simulink model "buoyancy_simulation"  (R2025a)
settings: Solver=VariableStepAuto  StartTime=0.0  StopTime=100  RelTol=1e-3
InitFcn:
  | parameters
values from neighbouring files (symbols this model uses):
  area = pi*(d/2)^2    (= 0.00785398163397)    [parameters.m]    (also in simulation_matlab.m)
  density = 1000    [parameters.m]
  gravity = 9.81    [parameters.m]
  km = 50    [parameters.m]
  mass = 3    [parameters.m]
  p = 0.002    [parameters.m]    (also in simulation_matlab.m)
  surface_buoyancy = 2.94    [parameters.m]
libraries: slpidlib x1
settings Model: Creator=hannasennero  LastModifiedBy=hannasennero

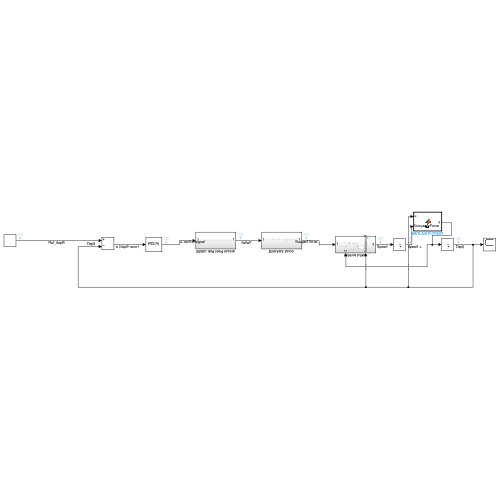
[thumbnail: Simulink's stored preview of the top-level diagram]
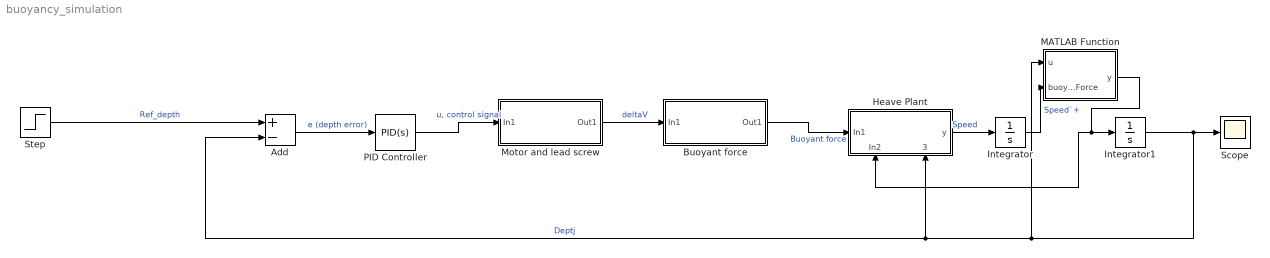
== system buoyancy_simulation ==
  Add : Sum  Inputs=+-
  Buoyant force : Subsystem
  Heave Plant : Subsystem
      settings: PortSchema="{\"entries\":[{\"content\":{\"sides\":[{\"content\":{\"connectorIds\":[\"In1\"]},\"type\":\"ConnectorPlacement.EquallySpacedRectSide\",\"uuid\":\"64163796-67b4-4874-a81c-abb8813ac274\"},{\"content\":{\"connectorIds\":[\"Out1\"],\"side\":\"RIGHT\"},\"type\":\"ConnectorPlacement.EquallySpacedRectSide\",\"uuid\":\"c10edb53-fdb3-4b5f-a96a-74da846fe7c3\"},{\"content\":{\"side\":\"TOP\"},\"type\":\"ConnectorPlacement.EquallySpacedRectSide\",\"uuid\":\"03a8d6bf-bc70-4644-992b-47d9b15e439c\"},{\"content\":{\"connectorIds\":[\"In2\",\"In3\"],\"side\":\"BOTTOM\"},\"type\":\"ConnectorPlacement.EquallySpacedRectSide\",\"uuid\":\"3bbf4b5d-45ae-4ac2-bdf5-5e5dee5a19eb\"}]},\"type\":\"ConnectorPlacement.EquallySpacedConnector\",\"uuid\":\"f3efd6ea-c772-4fc4-945d-e21c2b4b2ad1\"}],\"packageUris\":[\"http://schema.mathworks.com/mf0/Connector/R2020b\"],\"version\":\"1.0\"}"
  Integrator : Integrator
  Integrator1 : Integrator
  MATLAB Function : MATLAB Function  TreatAsAtomicUnit=on
  Motor and lead screw : Subsystem
  PID Controller : slpidlib/PID Controller  Controller=PID  Form=Parallel  TimeDomain=Continuous-time  UseExternalTs=off  SampleTime=-1  IntegratorMethod=Forward Euler  FilterMethod=Forward Euler  ControllerParametersSource=internal  P=5  I=0  UseKiTs=off  D=1  UseExternalDerivativeSource=off  N=100  UseFilter=on  TunerSelectOption=Transfer Function Based (PID Tuner App)  InitialConditionSource=internal  InitialConditionForIntegrator=0  InitialConditionForFilter=0  DifferentiatorICPrevScaledInput=0  ExternalReset=none  TrackingMode=off  Kt=1  LimitOutput=off  SatLimitsSource=internal  UpperSaturationLimit=inf  LowerSaturationLimit=-inf  LinearizeAsGain=on  AntiWindupMode=none  Kb=1  LimitIntegrator=off  UpperIntegratorSaturationLimit=inf  LowerIntegratorSaturationLimit=-inf  POutMin=[]  POutMax=[]  IOutMin=[]  IOutMax=[]  DOutMin=[]  DOutMax=[]  NOutMin=[]  NOutMax=[]  SumOutMin=[]  SumOutMax=[]  SaturationOutMin=[]  SaturationOutMax=[]  PParamMin=[]  PParamMax=[]  IParamMin=[]  IParamMax=[]  DParamMin=[]  DParamMax=[]  NParamMin=[]  NParamMax=[]  KbParamMin=[]  KbParamMax=[]  KtParamMin=[]  KtParamMax=[]  KbOutMin=[]  KbOutMax=[]  KtOutMin=[]  KtOutMax=[]  IntegratorOutMin=[]  IntegratorOutMax=[]  FilterOutMin=[]  FilterOutMax=[]  SumI1OutMin=[]  SumI1OutMax=[]  SumI2OutMin=[]  SumI2OutMax=[]  SumI3OutMin=[]  SumI3OutMax=[]  SumI4OutMin=[]  SumI4OutMax=[]  SumDOutMin=[]  SumDOutMax=[]  DifferentiatorOutMin=[]  DifferentiatorOutMax=[]  FilterDiffOutCoefMin=[]  FilterDiffOutCoefMax=[]  ReciprocalOutMin=[]  ReciprocalOutMax=[]  SumDenOutMin=[]  SumDenOutMax=[]  SumNumOutMin=[]  SumNumOutMax=[]  DivideOutMin=[]  DivideOutMax=[]  UdiffTsProdOutMin=[]  UdiffTsProdOutMax=[]  NTsProdOutMin=[]  NTsProdOutMax=[]  UintegralTsProdOutMin=[]  UintegralTsProdOutMax=[]  UngainTsProdOutMin=[]  UngainTsProdOutMax=[]  ClampingZeroOutDataTypeStr=Inherit: Inherit via back propagation  ClampingZeroOutMin=[]  ClampingZeroOutMax=[]  FilterDenConstantOutDataTypeStr=Inherit: Inherit via back propagation  FilterDenConstantOutMin=[]  FilterDenConstantOutMax=[]  PCopyOutDataTypeStr=Inherit: Inherit via back propagation  PCopyOutMin=[]  PCopyOutMax=[]  NCopyOutDataTypeStr=Inherit: Inherit via back propagation  NCopyOutMin=[]  NCopyOutMax=[]  IntegratorContinuousStateAttributes=''  IntegratorStateMustResolveToSignalObject=off  IntegratorRTWStateStorageClass=Auto  FilterContinuousStateAttributes=''  FilterStateMustResolveToSignalObject=off  FilterRTWStateStorageClass=Auto  ParallelPVariant=InternalParameters  IdealPVariant=Disabled  IVariant=InternalParameters  DVariant=InternalParameters  IntegratorVariant=Continuous  SatVariant=Disabled  AWVariant=Passthrough  PCopyVariant=Disabled  TRVariant=Disabled  FdbkBlocksVariant=Forward  IdealPFdbkVariant=Disabled  SatFdbkVariant=Disabled  DerivativeFilterVariant=ContFilter  NVariant=InternalParameters  NCopyVariant=Disabled  FilterICVariant=InternalICsFilter  IntegratorICVariant=InternalICs  ExternalResetVariant=Disabled  TRSumVariant=Passthrough  SumFdbkVariant=Disabled  SumVariant=Sum_PID  TsampFilterVariant=InternalTs  TsampNgainVariant=Passthrough  TsampIntegralVariant=Disabled_SignalSpec  ExternalSaturationOutDataTypeStr=Inherit: Same as second input  DerivativeSourceVariant=ErrorSignal  PreIntVariant=InternalPreInt
  Scope : Scope
      settings: ActiveDisplayYMinimum=-21.142736439512891  ActiveDisplayYMaximum=-18.092954060228088
  Step : Step  After=-3  SampleTime=0
  wires:
  Step/1 -> Add/1  "Ref_depth"
  Heave Plant/1(y) -> Integrator/1  "Speed"
  Add/1 -> PID Controller/1  "e (depth error)"
  PID Controller/1 -> Motor and lead screw/1(In1)  "u, control signal"
  Motor and lead screw/1(Out1) -> Buoyant force/1(In1)  "deltaV"
  Buoyant force/1(Out1) -> Heave Plant/1(In1)  "Buoyant force"
  Integrator/1 -> MATLAB Function/2(buoyancyForce)  "Speed`+"
  Integrator1/1 -> Scope/1, MATLAB Function/1(u), Heave Plant/3(buoyancyForce), Add/2  "Deptj"
  MATLAB Function/1(y) -> Integrator1/1, Heave Plant/2(In2)

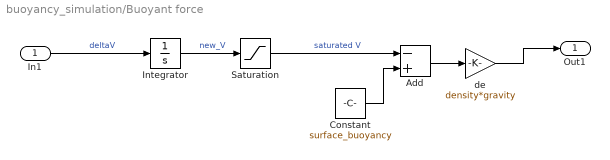
== system buoyancy_simulation/Buoyant force ==
  In1 : Inport
  Add : Sum  Inputs=-+
  Constant : Constant  Value=surface_buoyancy
  Integrator : Integrator
  Saturation : Saturate  UpperLimit=500  LowerLimit=-500
  de : Gain  Gain=density*gravity
  Out1 : Outport
  wires:
  In1/1 -> Integrator/1  "deltaV"
  Integrator/1 -> Saturation/1  "new_V"
  Add/1 -> de/1
  Constant/1 -> Add/2
  Saturation/1 -> Add/1  "saturated V"
  de/1 -> Out1/1

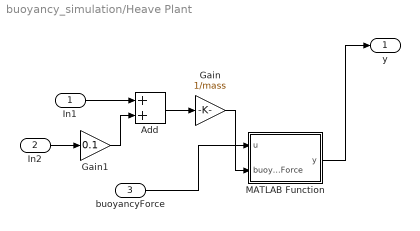
== system buoyancy_simulation/Heave Plant ==
  In1 : Inport
  In2 : Inport  Port=2
  buoyancyForce : Inport  Port=3
  Add : Sum
  Gain : Gain  Gain=1/mass
  Gain1 : Gain  Gain=0.1
  MATLAB Function : MATLAB Function  TreatAsAtomicUnit=on
  y : Outport
  wires:
  Add/1 -> Gain/1
  Gain1/1 -> Add/2
  In2/1 -> Gain1/1
  MATLAB Function/1(y) -> y/1
  buoyancyForce/1 -> MATLAB Function/1(u)
  Gain/1 -> MATLAB Function/2(buoyancyForce)
  In1/1 -> Add/1

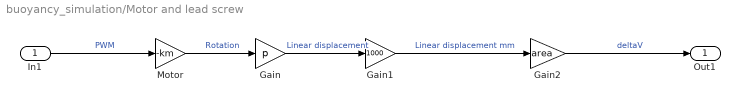
== system buoyancy_simulation/Motor and lead screw ==
  In1 : Inport
  Gain : Gain  Gain=p
  Gain1 : Gain  Gain=1000
  Gain2 : Gain  Gain=area
  Motor : Gain  Gain=-km
  Out1 : Outport
  wires:
  In1/1 -> Motor/1  "PWM"
  Motor/1 -> Gain/1  "Rotation"
  Gain/1 -> Gain1/1  "Linear displacement"
  Gain2/1 -> Out1/1  "deltaV"
  Gain1/1 -> Gain2/1  "Linear displacement mm"

== matlab function buoyancy_simulation/Heave Plant/MATLAB Function ==
  data: u input; y output; buoyancyForce input
function y = fcn(u, buoyancyForce)
    if u > 0.1 && buoyancyForce > 0
        y = 0;
    else
        y = buoyancyForce;
    end
end

== matlab function buoyancy_simulation/MATLAB Function ==
  data: u input; y output; buoyancyForce input
function y = fcn(u, buoyancyForce)
    if u > 0.1 && buoyancyForce > 0
        y = 0;
    else
        y = buoyancyForce;
    end
end
